simulink model "Magnetic_levitation"  (R2024a)
settings: Solver=VariableStepAuto  StartTime=0.0  StopTime=10.0  RelTol=1e-3
values from neighbouring files (symbols this model uses):
  f1max = (g*mu*(mu*-0.3+2*mu*zref+2))/((1+mu*(zref-0.3))^2)    (= 132.708333333)    [Controldesign_Magnetic_levitation.m]
  f1min = (g*mu*(mu*0.3+2*mu*zref+2))/((1+mu*(zref+0.3))^2)    (= 19.1666666667)    [Controldesign_Magnetic_levitation.m]
  f2max = (-lambda*mu)/(2*m*(1+mu*(zref+0.3))^2)    [Controldesign_Magnetic_levitation.m]
  f2min = (-lambda*mu)/(2*m*(1+mu*(zref-0.3))^2)    [Controldesign_Magnetic_levitation.m]
  g = 9.8    [Controldesign_Magnetic_levitation.m]
  iref2 = (2*m*g*(1+mu*zref)^2)/(lambda*mu)    [Controldesign_Magnetic_levitation.m]
  K11 = value(K{1}{1})    [Controldesign_Magnetic_levitation.m]
  K12 = value(K{1}{2})    [Controldesign_Magnetic_levitation.m]
  K13 = value(K{1}{3})    [Controldesign_Magnetic_levitation.m]
  K14 = value(K{1}{4})    [Controldesign_Magnetic_levitation.m]
  K21 = value(K{2}{1})    [Controldesign_Magnetic_levitation.m]
  K22 = value(K{2}{2})    [Controldesign_Magnetic_levitation.m]
  K23 = value(K{2}{3})    [Controldesign_Magnetic_levitation.m]
  K24 = value(K{2}{4})    [Controldesign_Magnetic_levitation.m]
  K31 = value(K{3}{1})    [Controldesign_Magnetic_levitation.m]
  K32 = value(K{3}{2})    [Controldesign_Magnetic_levitation.m]
  K33 = value(K{3}{3})    [Controldesign_Magnetic_levitation.m]
  K34 = value(K{3}{4})    [Controldesign_Magnetic_levitation.m]
  K41 = value(K{4}{1})    [Controldesign_Magnetic_levitation.m]
  K42 = value(K{4}{2})    [Controldesign_Magnetic_levitation.m]
  K43 = value(K{4}{3})    [Controldesign_Magnetic_levitation.m]
  K44 = value(K{4}{4})    [Controldesign_Magnetic_levitation.m]
  kk = 0.001    [Controldesign_Magnetic_levitation.m]
  lambda = 0.46    [Controldesign_Magnetic_levitation.m]
  m = 0.05    [Controldesign_Magnetic_levitation.m]    (also in Theorem_2.m = length(B{1}(1,:)))
  mm = length(B{1}(1,:))    [Controldesign_Magnetic_levitation.m]
  mu = 2    [Controldesign_Magnetic_levitation.m]
  P1 = value(P{1})    [Controldesign_Magnetic_levitation.m]
  P2 = value(P{2})    [Controldesign_Magnetic_levitation.m]
  P3 = value(P{3})    [Controldesign_Magnetic_levitation.m]
  P4 = value(P{4})    [Controldesign_Magnetic_levitation.m]
  zref = 0.04    [Controldesign_Magnetic_levitation.m]
settings Model: Creator=dante  LastModifiedBy=dante
settings DataIOCC: InitialState=IC  LoadInitialState=on  ReturnWorkspaceOutputs=off

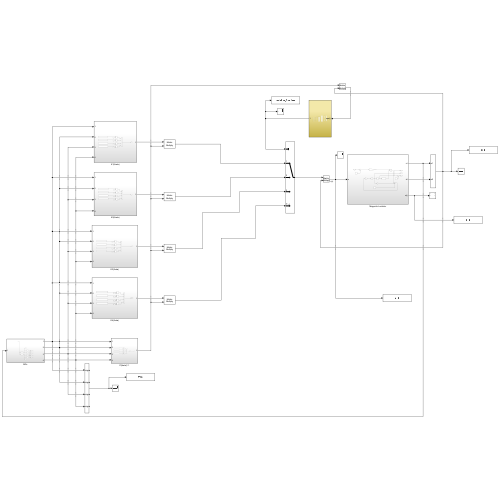
[thumbnail: Simulink's stored preview of the top-level diagram]
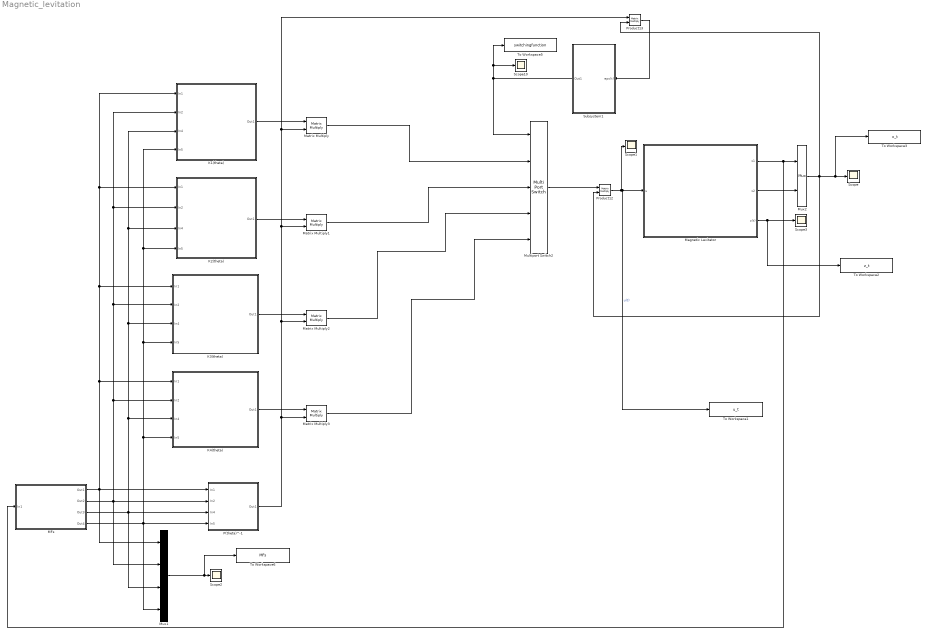
== system Magnetic_levitation ==
  K1(theta) : Subsystem
  K2(theta) : Subsystem
  K3(theta) : Subsystem
  K4(theta) : Subsystem
  "MFs " : Subsystem
  Magnetic Levitator : Subsystem
  Matrix Multiply{,1..3} (4 alike) : Product  Multiplication=Matrix(*)
  Multiport Switch2 : MultiPortSwitch  Inputs=4  SaturateOnIntegerOverflow=off  InputSameDT=off
  Mux1 : Mux
      settings: DisplayOption=signals
  Mux2 : Mux  Inputs=2
      settings: DisplayOption=signals
  P(theta)^-1 : Subsystem
  Product12 : Product  Multiplication=Matrix(*)
  Product13 : Product  Multiplication=Matrix(*)
  Scope{,1..3,10} (5 alike) : Scope
  Subsystem1 : Subsystem
  To Workspace1 : ToWorkspace  VariableName=u_t  SampleTime=-1
  To Workspace2 : ToWorkspace  VariableName=z_t  SampleTime=-1
  To Workspace3 : ToWorkspace  VariableName=x_t  SampleTime=-1
  To Workspace5 : ToWorkspace  VariableName=switchingfunction  SampleTime=-1
  To Workspace6 : ToWorkspace  VariableName=MFs  SampleTime=-1
  wires:
  Product12/1 -> To Workspace1/1, Magnetic Levitator/1(u), Scope1/1  "u(t)"
  Multiport Switch2/1 -> Product12/1
  Magnetic Levitator/1(x1) -> Mux2/1, "MFs "/1(In1)
  Subsystem1/1(Out1) -> Multiport Switch2/1, To Workspace5/1, Scope10/1
  Product13/1 -> Subsystem1/1(eps(t))
  P(theta)^-1/1(Out1) -> Matrix Multiply3/2, Matrix Multiply1/2, Product13/1, Matrix Multiply/2, Matrix Multiply2/2
  Mux2/1 -> Product12/2, To Workspace3/1, Scope/1, Product13/2
  "MFs "/2(Out2) -> Mux1/2, P(theta)^-1/2(In2), K3(theta)/2(In2), K2(theta)/2(In2), K1(theta)/2(In2), K4(theta)/2(In2)
  "MFs "/3(Out3) -> Mux1/3, K4(theta)/3(In4), K3(theta)/3(In4), K2(theta)/3(In4), K1(theta)/3(In4), P(theta)^-1/3(In4)
  "MFs "/4(Out4) -> P(theta)^-1/4(In5), Mux1/4, K4(theta)/4(In5), K3(theta)/4(In5), K2(theta)/4(In5), K1(theta)/4(In5)
  "MFs "/1(Out1) -> Mux1/1, K4(theta)/1(In1), K3(theta)/1(In1), K2(theta)/1(In1), K1(theta)/1(In1), P(theta)^-1/1(In1)
  K1(theta)/1(Out1) -> Matrix Multiply/1
  K2(theta)/1(Out1) -> Matrix Multiply1/1
  K3(theta)/1(Out1) -> Matrix Multiply2/1
  K4(theta)/1(Out1) -> Matrix Multiply3/1
  Matrix Multiply/1 -> Multiport Switch2/2
  Matrix Multiply1/1 -> Multiport Switch2/3
  Matrix Multiply2/1 -> Multiport Switch2/4
  Matrix Multiply3/1 -> Multiport Switch2/5
  Mux1/1 -> To Workspace6/1, Scope2/1
  Magnetic Levitator/2(x2) -> Mux2/2
  Magnetic Levitator/3(z(t)) -> To Workspace2/1, Scope3/1

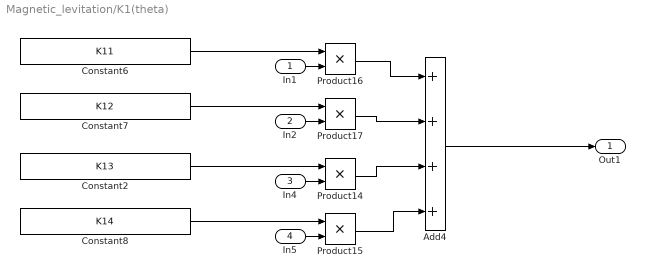
== system Magnetic_levitation/K1(theta) ==
  In1 : Inport
  In2 : Inport  Port=2
  In4 : Inport  Port=3
  In5 : Inport  Port=4
  Add4 : Sum  Inputs=++++
  Constant2 : Constant  Value=K13
  Constant6 : Constant  Value=K11
  Constant7 : Constant  Value=K12
  Constant8 : Constant  Value=K14
  Product{14..17} (4 alike) : Product
  Out1 : Outport
  wires:
  Product15/1 -> Add4/4
  Constant8/1 -> Product15/1
  Product16/1 -> Add4/1
  Constant7/1 -> Product17/1
  In4/1 -> Product14/2
  Constant6/1 -> Product16/1
  Product17/1 -> Add4/2
  Product14/1 -> Add4/3
  Constant2/1 -> Product14/1
  In5/1 -> Product15/2
  In2/1 -> Product17/2
  In1/1 -> Product16/2
  Add4/1 -> Out1/1

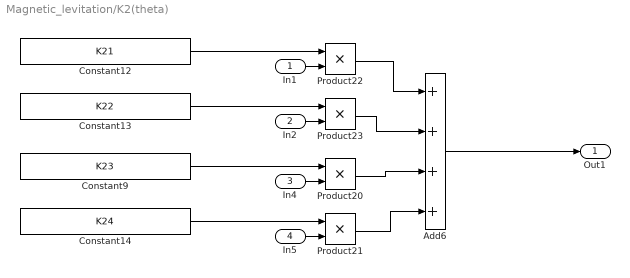
== system Magnetic_levitation/K2(theta) ==
  In1 : Inport
  In2 : Inport  Port=2
  In4 : Inport  Port=3
  In5 : Inport  Port=4
  Add6 : Sum  Inputs=++++
  Constant12 : Constant  Value=K21
  Constant13 : Constant  Value=K22
  Constant14 : Constant  Value=K24
  Constant9 : Constant  Value=K23
  Product{20..23} (4 alike) : Product
  Out1 : Outport
  wires:
  Constant14/1 -> Product21/1
  In5/1 -> Product21/2
  Constant9/1 -> Product20/1
  Product23/1 -> Add6/2
  Product22/1 -> Add6/1
  Constant12/1 -> Product22/1
  Add6/1 -> Out1/1
  Constant13/1 -> Product23/1
  Product20/1 -> Add6/3
  In4/1 -> Product20/2
  Product21/1 -> Add6/4
  In2/1 -> Product23/2
  In1/1 -> Product22/2

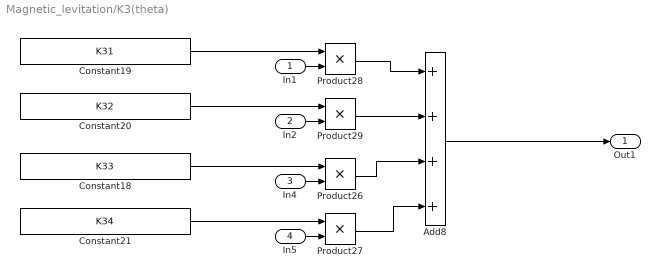
== system Magnetic_levitation/K3(theta) ==
  In1 : Inport
  In2 : Inport  Port=2
  In4 : Inport  Port=3
  In5 : Inport  Port=4
  Add8 : Sum  Inputs=++++
  Constant18 : Constant  Value=K33
  Constant19 : Constant  Value=K31
  Constant20 : Constant  Value=K32
  Constant21 : Constant  Value=K34
  Product{26..29} (4 alike) : Product
  Out1 : Outport
  wires:
  Product29/1 -> Add8/2
  Constant18/1 -> Product26/1
  Product26/1 -> Add8/3
  Product28/1 -> Add8/1
  Product27/1 -> Add8/4
  Constant19/1 -> Product28/1
  Constant20/1 -> Product29/1
  Constant21/1 -> Product27/1
  In5/1 -> Product27/2
  In1/1 -> Product28/2
  In2/1 -> Product29/2
  In4/1 -> Product26/2
  Add8/1 -> Out1/1

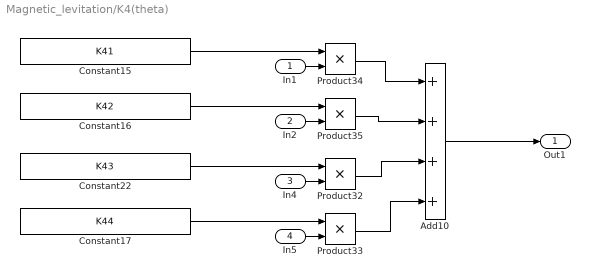
== system Magnetic_levitation/K4(theta) ==
  In1 : Inport
  In2 : Inport  Port=2
  In4 : Inport  Port=3
  In5 : Inport  Port=4
  Add10 : Sum  Inputs=++++
  Constant15 : Constant  Value=K41
  Constant16 : Constant  Value=K42
  Constant17 : Constant  Value=K44
  Constant22 : Constant  Value=K43
  Product{32..35} (4 alike) : Product
  Out1 : Outport
  wires:
  Constant16/1 -> Product35/1
  Constant22/1 -> Product32/1
  Product35/1 -> Add10/2
  In2/1 -> Product35/2
  Product33/1 -> Add10/4
  Product32/1 -> Add10/3
  Product34/1 -> Add10/1
  Constant15/1 -> Product34/1
  Constant17/1 -> Product33/1
  In5/1 -> Product33/2
  In1/1 -> Product34/2
  In4/1 -> Product32/2
  Add10/1 -> Out1/1

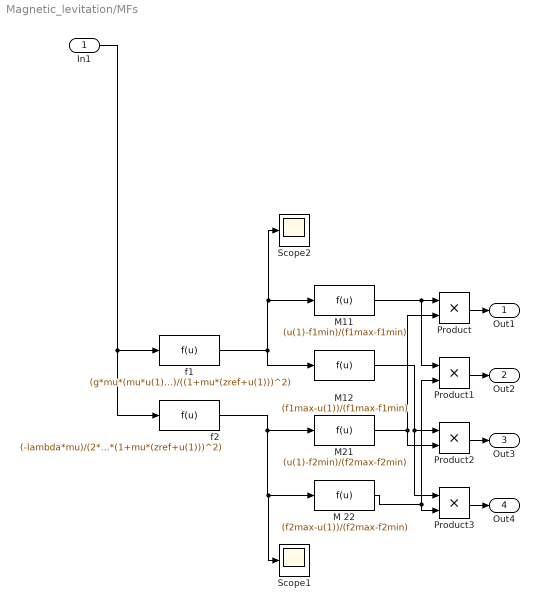
== system Magnetic_levitation/MFs  ==
  In1 : Inport
  M 22 : Fcn  Expr=(f2max-u(1))/(f2max-f2min)
  M11 : Fcn  Expr=(u(1)-f1min)/(f1max-f1min)
  M12 : Fcn  Expr=(f1max-u(1))/(f1max-f1min)
  M21 : Fcn  Expr=(u(1)-f2min)/(f2max-f2min)
  Product{,1..3} (4 alike) : Product
  Scope1 : Scope
  Scope2 : Scope
  f1 : Fcn  Expr=(g*mu*(mu*u(1)+2*mu*zref+2))/((1+mu*(zref+u(1)))^2)
  f2 : Fcn  Expr=(-lambda*mu)/(2*mm*(1+mu*(zref+u(1)))^2)
  Out1 : Outport
  Out2 : Outport  Port=2
  Out3 : Outport  Port=3
  Out4 : Outport  Port=4
  wires:
  f1/1 -> M12/1, Scope2/1, M11/1
  f2/1 -> Scope1/1, M 22/1, M21/1
  M21/1 -> Product/2, Product2/2
  M11/1 -> Product1/1, Product/1
  M 22/1 -> Product1/2, Product3/2
  Product1/1 -> Out2/1
  Product3/1 -> Out4/1
  In1/1 -> f2/1, f1/1
  M12/1 -> Product3/1, Product2/1
  Product/1 -> Out1/1
  Product2/1 -> Out3/1

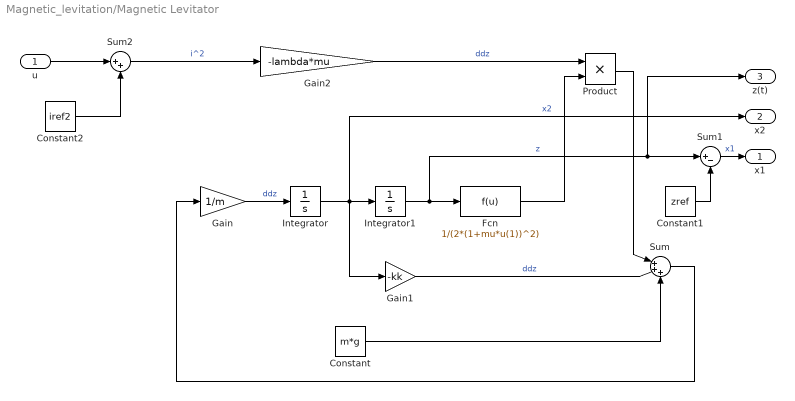
== system Magnetic_levitation/Magnetic Levitator ==
  u : Inport
  Constant : Constant  Value=m*g
  Constant1 : Constant  Value=zref
  Constant2 : Constant  Value=iref2
  Fcn : Fcn  Expr=1/(2*(1+mu*u(1))^2)
  Gain : Gain  Gain=1/m
  Gain1 : Gain  Gain=-kk
  Gain2 : Gain  Gain=-lambda*mu
  Integrator : Integrator
  Integrator1 : Integrator
  Product : Product
  Sum : Sum  Inputs=|+++
  Sum1 : Sum  Inputs=|+-
  Sum2 : Sum  Inputs=|++
  x1 : Outport
  x2 : Outport  Port=2
  z(t) : Outport  Port=3
  wires:
  Constant/1 -> Sum/3
  Gain/1 -> Integrator/1  "ddz"
  Integrator/1 -> x2/1, Gain1/1, Integrator1/1  "x2"
  Fcn/1 -> Product/2
  Integrator1/1 -> z(t)/1, Sum1/1, Fcn/1  "z"
  Gain1/1 -> Sum/2  "ddz"
  Gain2/1 -> Product/1  "ddz"
  Product/1 -> Sum/1
  Sum/1 -> Gain/1
  Sum1/1 -> x1/1  "x1"
  Constant1/1 -> Sum1/2
  u/1 -> Sum2/1
  Constant2/1 -> Sum2/2
  Sum2/1 -> Gain2/1  "i^2"

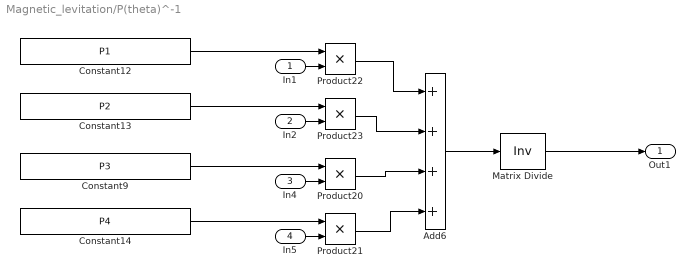
== system Magnetic_levitation/P(theta)^-1 ==
  In1 : Inport
  In2 : Inport  Port=2
  In4 : Inport  Port=3
  In5 : Inport  Port=4
  Add6 : Sum  Inputs=++++
  Constant12 : Constant  Value=P1
  Constant13 : Constant  Value=P2
  Constant14 : Constant  Value=P4
  Constant9 : Constant  Value=P3
  Matrix Divide : Product  Inputs=/  Multiplication=Matrix(*)
  Product{20..23} (4 alike) : Product
  Out1 : Outport
  wires:
  Constant14/1 -> Product21/1
  In5/1 -> Product21/2
  Constant9/1 -> Product20/1
  Product23/1 -> Add6/2
  Product22/1 -> Add6/1
  Constant12/1 -> Product22/1
  Add6/1 -> Matrix Divide/1
  Matrix Divide/1 -> Out1/1
  Constant13/1 -> Product23/1
  Product20/1 -> Add6/3
  In4/1 -> Product20/2
  Product21/1 -> Add6/4
  In2/1 -> Product23/2
  In1/1 -> Product22/2

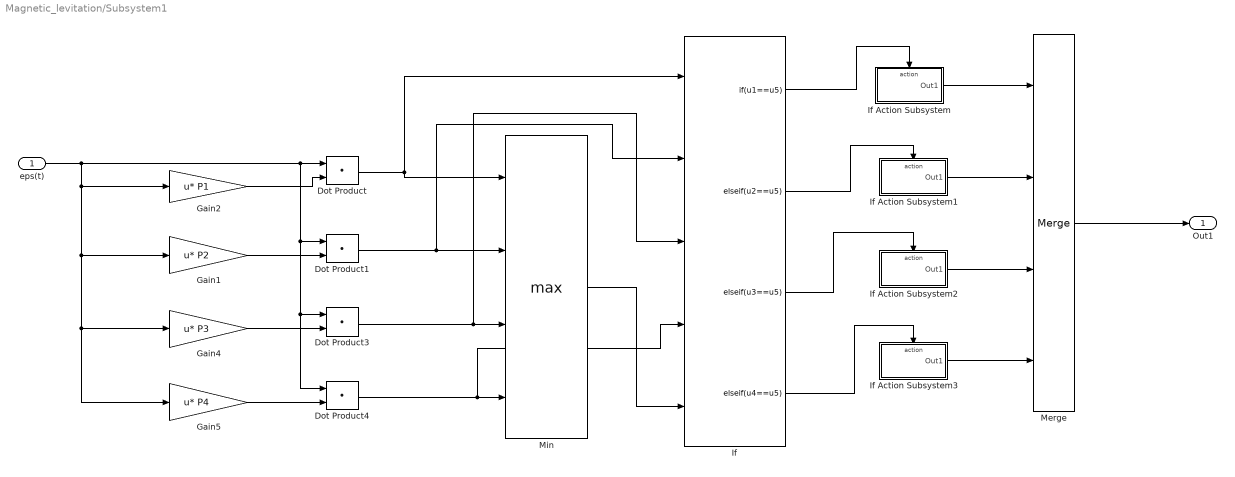
== system Magnetic_levitation/Subsystem1 ==
  eps(t) : Inport
  Dot Product{,1,3..4} (4 alike) : DotProduct  OutDataTypeStr=Inherit: Inherit via internal rule
  Gain1 : Gain  Gain=P2  Multiplication=Matrix(u*K)
  Gain2 : Gain  Gain=P1  Multiplication=Matrix(u*K)
  Gain4 : Gain  Gain=P3  Multiplication=Matrix(u*K)
  Gain5 : Gain  Gain=P4  Multiplication=Matrix(u*K)
  If : If  NumInputs=5  IfExpression=u1==u5  ElseIfExpressions=u2==u5, u3==u5,u4==u5  ShowElse=off  ZeroCross=off
  If Action Subsystem : Subsystem  TreatAsAtomicUnit=on
  If Action Subsystem1 : Subsystem  TreatAsAtomicUnit=on
  If Action Subsystem2 : Subsystem  TreatAsAtomicUnit=on
  If Action Subsystem3 : Subsystem  TreatAsAtomicUnit=on
  Merge : Merge  Inputs=4
  Min : MinMax  Function=max  Inputs=4  ZeroCross=off
  Out1 : Outport
  wires:
  If/1 -> If Action Subsystem/Action
  If Action Subsystem/1(Out1) -> Merge/1
  If/2 -> If Action Subsystem1/Action
  Merge/1 -> Out1/1
  Dot Product/1 -> If/1, Min/1
  Dot Product1/1 -> If/2, Min/2
  Gain2/1 -> Dot Product/2
  Gain1/1 -> Dot Product1/2
  eps(t)/1 -> Gain4/1, Gain5/1, Gain1/1, Gain2/1, Dot Product4/1, Dot Product3/1, Dot Product1/1, Dot Product/1
  Gain5/1 -> Dot Product4/2
  Gain4/1 -> Dot Product3/2
  Dot Product3/1 -> If/3, Min/3
  Dot Product4/1 -> If/4, Min/4
  Min/1 -> If/5
  If/3 -> If Action Subsystem2/Action
  If/4 -> If Action Subsystem3/Action
  If Action Subsystem1/1(Out1) -> Merge/2
  If Action Subsystem2/1(Out1) -> Merge/3
  If Action Subsystem3/1(Out1) -> Merge/4

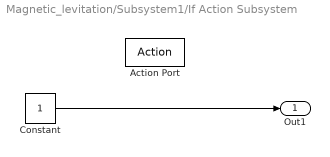
== system Magnetic_levitation/Subsystem1/If Action Subsystem ==
  Action Port : ActionPort  ActionPortLabel=if(u1==u5)
  Constant : Constant
  Out1 : Outport
  wires:
  Constant/1 -> Out1/1

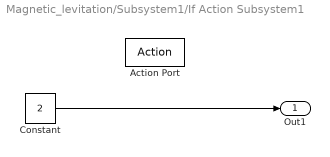
== system Magnetic_levitation/Subsystem1/If Action Subsystem1 ==
  Action Port : ActionPort  ActionPortLabel=elseif(u2==u5)
  Constant : Constant  Value=2
  Out1 : Outport
  wires:
  Constant/1 -> Out1/1

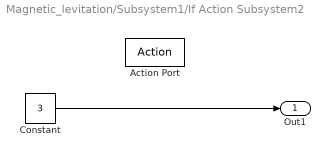
== system Magnetic_levitation/Subsystem1/If Action Subsystem2 ==
  Action Port : ActionPort  ActionPortLabel=elseif( u3==u5)
  Constant : Constant  Value=3
  Out1 : Outport
  wires:
  Constant/1 -> Out1/1

== system Magnetic_levitation/Subsystem1/If Action Subsystem3 ==
  Action Port : ActionPort  ActionPortLabel=elseif(u4==u5)
  Constant : Constant  Value=4
  Out1 : Outport
  wires:
  Constant/1 -> Out1/1
